simulink model "PID"  (R2018b)
settings: Solver=FixedStepAuto  StartTime=0.0  StopTime=7  RelTol=1e-3
values from neighbouring files (symbols this model uses):
  cond_init = [x1,x2,x3,x4,x5,x6]'    [main.m]
  Law = [100,5]    [main.m]
  param = param'    [main.m]
  Ts = 0.1    [find_solution_joint.m]    (also in main.m = 0.05)
undefined symbols (not defined in the file or in its folder): pos
settings Model: Creator=AmatoPi  LastModifiedBy=Utente

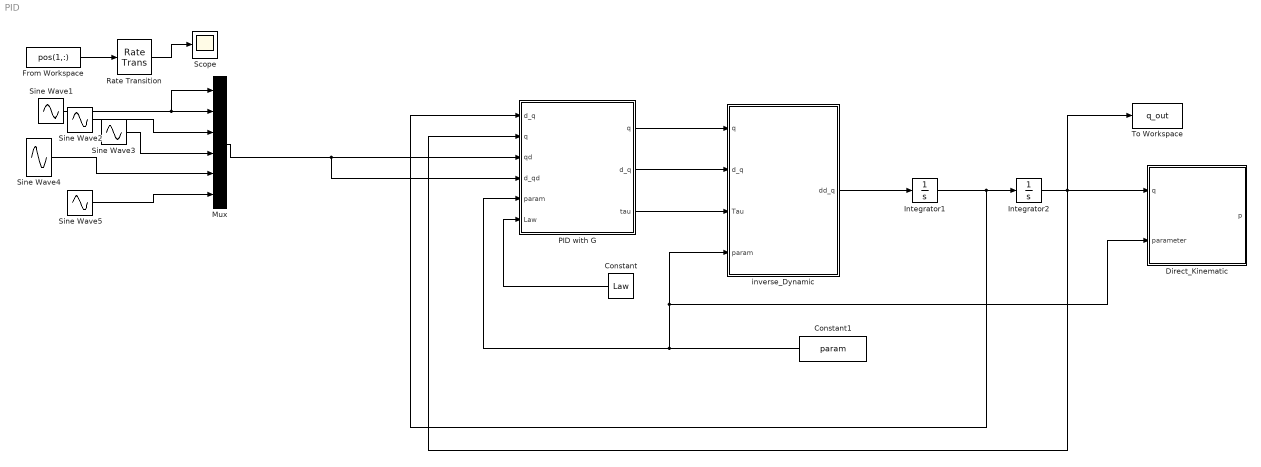
== system PID ==
  Constant : Constant  Value=Law
  Constant1 : Constant  Value=param
  Direct_Kinematic : MATLAB Function  TreatAsAtomicUnit=on
  From Workspace : FromWorkspace  VariableName=pos(1,:)  OutDataTypeStr=double  SampleTime=Ts  OutputAfterFinalValue=Holding final value
  Integrator1 : Integrator  InitialCondition=[0;0;0;0;0;0]
  Integrator2 : Integrator  InitialCondition=cond_init
  Mux : Mux  Inputs=6
  PID with G : MATLAB Function  TreatAsAtomicUnit=on
  Rate Transition : RateTransition  InitialCondition=pos(1,1)  OutPortSampleTimeOpt=Multiple of input port sample time  OutPortSampleTimeMultiple=Ts  OutPortSampleTime=Ts
  Scope : Scope
  Sine Wave{1..5} (5 alike) : Sin  SampleTime=0
  To Workspace : ToWorkspace  VariableName=q_out  SaveFormat=Timeseries  SampleTime=-1
  inverse_Dynamic : MATLAB Function  TreatAsAtomicUnit=on
  wires:
  PID with G/3(tau) -> inverse_Dynamic/3(Tau)
  PID with G/2(d_q) -> inverse_Dynamic/2(d_q)
  PID with G/1(q) -> inverse_Dynamic/1(q)
  inverse_Dynamic/1(dd_q) -> Integrator1/1
  Integrator1/1 -> PID with G/1("d_q "), Integrator2/1
  Integrator2/1 -> Direct_Kinematic/1(q), To Workspace/1, PID with G/2("q ")
  Constant/1 -> PID with G/6(Law)
  Constant1/1 -> PID with G/5(param), Direct_Kinematic/2(parameter), inverse_Dynamic/4(param)
  Sine Wave2/1 -> Mux/3
  Sine Wave3/1 -> Mux/4
  Sine Wave4/1 -> Mux/5
  Sine Wave5/1 -> Mux/6
  Mux/1 -> PID with G/4(d_qd), PID with G/3(qd)
  From Workspace/1 -> Rate Transition/1
  Sine Wave1/1 -> Mux/1, Mux/2
  Rate Transition/1 -> Scope/1

== matlab function PID/PID with G ==
  data: q output; d_q output; d_q input; tau output; q input; qd input; d_qd input; param input; Law input
function [q,d_q,tau]  = PID_Contro(d_q, q, qd, d_qd, param, Law)

    kp = Law(1).*eye(6);
    kd = Law(2).*eye(6);
    [~,~,G] = Dinamica(param,q,d_q);
    
    error = qd - q;
    %d_error = d_qd - d_q;
    
    tau = kp*error + G % + kd*d_error ;
    
end

== matlab function PID/inverse_Dynamic ==
  data: q input; dd_q output; d_q input; Tau input; param input
function dd_q = inverseDynamic(q,d_q,Tau,param)
    
    [B,C,G] = Dinamica(param,q,d_q);

    tot = Tau - C*d_q - G;    
    dd_q = B\(tot);

end

== matlab function PID/Direct_Kinematic ==
  data: q input; p output; parameter input
function p = DirectK(q,parameter)

	[p,com,head] = Direct_Kinematics(parameter,q);
    
    

end
